simulink model "Metrics"  (R2024b)
settings: Solver=VariableStepAuto  StartTime=0.0  StopTime=10.0  RelTol=1e-3
settings Model: Creator=ryandavis  LastModifiedBy=ryandavis

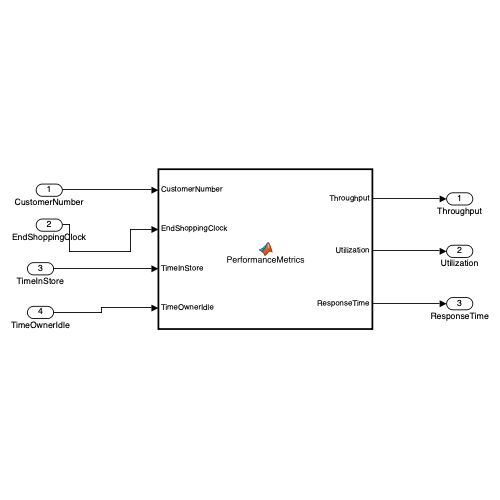
[thumbnail: Simulink's stored preview of the top-level diagram]
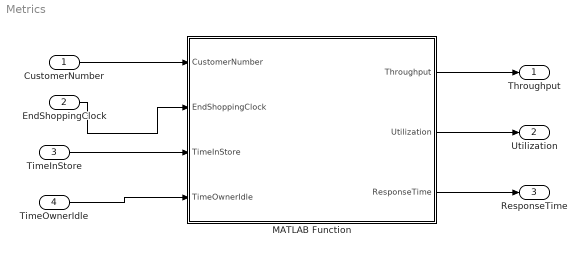
== system Metrics ==
  CustomerNumber : Inport
  EndShoppingClock : Inport  Port=2
  TimeInStore : Inport  Port=3
  TimeOwnerIdle : Inport  Port=4
  MATLAB Function : MATLAB Function  TreatAsAtomicUnit=on
  Throughput : Outport
  Utilization : Outport  Port=2
  ResponseTime : Outport  Port=3
  wires:
  MATLAB Function/1(Throughput) -> Throughput/1
  MATLAB Function/2(Utilization) -> Utilization/1
  MATLAB Function/3(ResponseTime) -> ResponseTime/1
  CustomerNumber/1 -> MATLAB Function/1(CustomerNumber)
  EndShoppingClock/1 -> MATLAB Function/2(EndShoppingClock)
  TimeInStore/1 -> MATLAB Function/3(TimeInStore)
  TimeOwnerIdle/1 -> MATLAB Function/4(TimeOwnerIdle)

== matlab function Metrics/MATLAB Function ==
  data: CustomerNumber input; Throughput output; EndShoppingClock input; TimeInStore input; TimeOwnerIdle input; Utilization output; ResponseTime output
function [Throughput, Utilization, ResponseTime] = PerformanceMetrics(CustomerNumber, EndShoppingClock, TimeInStore, TimeOwnerIdle)
    ObservedTime = CustomerNumber;
    
    Throughput = CustomerNumber / ObservedTime;
    
    TotalBusyTime = sum(EndShoppingClock) - TimeOwnerIdle;
    
    Utilization = (TotalBusyTime / ObservedTime) * 100;
    
    if CustomerNumber > 0
        ResponseTime = sum(TimeInStore) / CustomerNumber;
    else
        ResponseTime = 0;
    end
end
